simulink model "washou4"  (R2018b)
settings: Solver=VariableStepAuto  StartTime=0.0  StopTime=50  RelTol=1e-3
libraries: fuzblock x1
settings Model: Creator=15705  LastModifiedBy=15705

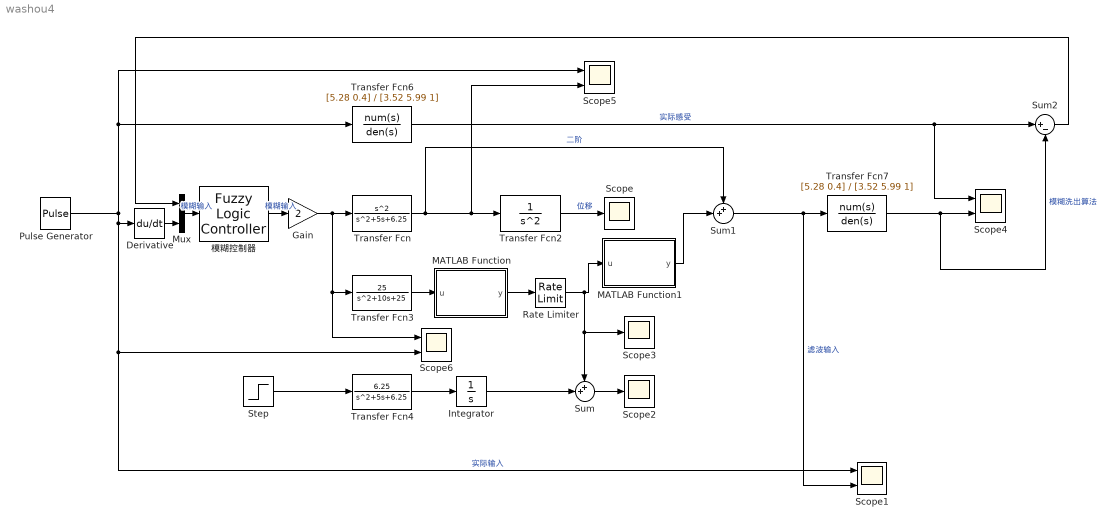
== system washou4 ==
  Derivative : Derivative
  Gain : Gain  Gain=2
  Integrator : Integrator
  MATLAB Function : MATLAB Function  TreatAsAtomicUnit=on
  MATLAB Function1 : MATLAB Function  TreatAsAtomicUnit=on
  Mux : Mux  Inputs=2
  Pulse Generator : DiscretePulseGenerator  PulseType=Time based  Period=20  PulseWidth=50  PhaseDelay=10
  Rate Limiter : RateLimiter  RisingSlewLimit=0.0628  FallingSlewLimit=-0.0628  SampleTimeMode=inherited
  Scope : Scope
  Scope{1,4..6} (4 alike) : Scope  NumInputPorts=2
  Scope2 : Scope
  Scope3 : Scope
  Step : Step  SampleTime=0
  Sum : Sum  Inputs=++|
  Sum1 : Sum  Inputs=++|
  Sum2 : Sum  Inputs=|+-
  Transfer Fcn : TransferFcn  Numerator=[1 0 0]  Denominator=[1 5 6.25]
  Transfer Fcn2 : TransferFcn  Denominator=[1 0 0]
  Transfer Fcn3 : TransferFcn  Numerator=[25]  Denominator=[1 10 25]
  Transfer Fcn4 : TransferFcn  Numerator=[6.25]  Denominator=[1 5 6.25]
  Transfer Fcn6 : TransferFcn  Numerator=[5.28 0.4]  Denominator=[3.52 5.99 1]
  Transfer Fcn7 : TransferFcn  Numerator=[5.28 0.4]  Denominator=[3.52 5.99 1]
  模糊控制器 : fuzblock/Fuzzy Logic  Controller  FIS=InputFuzzy  OutputSampleNumber=101  DataType=double  FuzzifiedInputs=off  RuleFiringStrengths=off  RuleOutputs=off  AggregatedOutputs=off  SimulateUsing=Interpreted execution  OutOfRangeInputValueMessage=warning  NoRuleFiredMessage=warning  EmptyOutputFuzzySetMessage=warning
  wires:
  Transfer Fcn/1 -> Scope5/2, Transfer Fcn2/1, Sum1/1  "二阶"
  Sum1/1 -> Scope1/2, Transfer Fcn7/1  "滤波输入"
  Transfer Fcn4/1 -> Integrator/1
  MATLAB Function1/1(y) -> Sum1/2
  Integrator/1 -> Sum/2
  Transfer Fcn3/1 -> MATLAB Function/1(u)
  Sum/1 -> Scope2/1
  Rate Limiter/1 -> MATLAB Function1/1(u), Scope3/1, Sum/1
  Transfer Fcn6/1 -> Sum2/1, Scope4/1  "实际感受"
  MATLAB Function/1(y) -> Rate Limiter/1
  Pulse Generator/1 -> Derivative/1, Scope6/2, Scope1/1, Transfer Fcn6/1, Scope5/1  "实际输入"
  Transfer Fcn2/1 -> Scope/1  "位移"
  Transfer Fcn7/1 -> Sum2/2, Scope4/2  "模糊洗出算法"
  Step/1 -> Transfer Fcn4/1
  模糊控制器/1 -> Gain/1  "模糊输入"
  Mux/1 -> 模糊控制器/1  "模糊输入"
  Derivative/1 -> Mux/2
  Sum2/1 -> Mux/1
  Gain/1 -> Transfer Fcn3/1, Scope6/1, Transfer Fcn/1

== matlab function washou4/MATLAB Function1 ==
  data: u input; y output
function y = fcn(u)
y=9.8*sin(u);

== matlab function washou4/MATLAB Function ==
  data: u input; y output
function y = fcn(u)
y=asin(u/9.8);
